simulink library "soar_lib"  (R2018b)
settings: Solver=VariableStepAuto  StartTime=0.0  StopTime=10.0  RelTol=1e-3
settings Model: Creator=Taylor  LastModifiedBy=Taylor
settings SFSimCC: SimUseLocalCustomCode=off
settings RTWCC: RTWUseLocalCustomCode=off
settings CodeAppCC: StateflowObjectComments=on

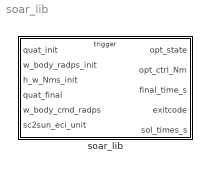
== system soar_lib ==
  soar_lib : Subsystem

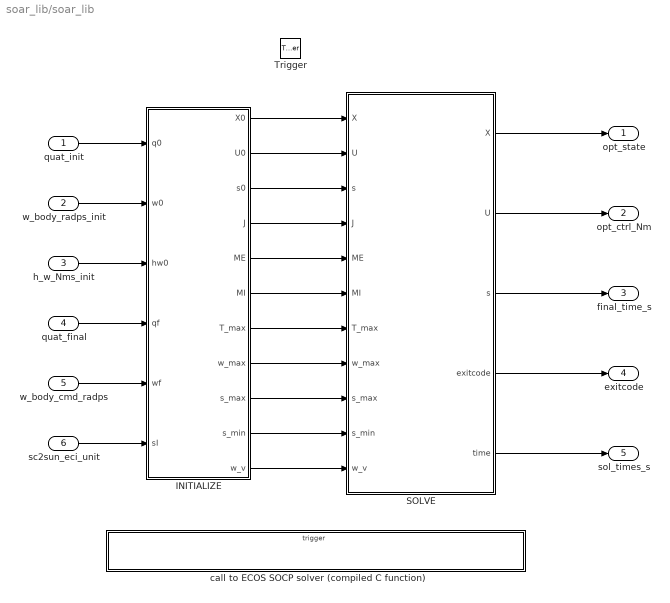
== system soar_lib/soar_lib ==
  quat_init : Inport
  w_body_radps_init : Inport  Port=2
  h_w_Nms_init : Inport  Port=3
  quat_final : Inport  Port=4
  w_body_cmd_radps : Inport  Port=5
  sc2sun_eci_unit : Inport  Port=6
  Trigger : TriggerPort  VariantControl=Variant  StatesWhenEnabling=reset  ZeroCross=off  InitialTriggerSignalState=zero  PortDimensions=1
  INITIALIZE : MATLAB Function  TreatAsAtomicUnit=on
  SOLVE : MATLAB Function  TreatAsAtomicUnit=on
  call to ECOS SOCP solver (compiled C function) : Subsystem  TreatAsAtomicUnit=on
  opt_state : Outport
  opt_ctrl_Nm : Outport  Port=2
  final_time_s : Outport  Port=3
  exitcode : Outport  Port=4
  sol_times_s : Outport  Port=5
  wires:
  h_w_Nms_init/1 -> INITIALIZE/3(hw0)
  sc2sun_eci_unit/1 -> INITIALIZE/6(sI)
  w_body_cmd_radps/1 -> INITIALIZE/5(wf)
  quat_final/1 -> INITIALIZE/4(qf)
  w_body_radps_init/1 -> INITIALIZE/2(w0)
  quat_init/1 -> INITIALIZE/1(q0)
  INITIALIZE/1(X0) -> SOLVE/1("X ")
  INITIALIZE/11(w_v) -> SOLVE/11(w_v)
  INITIALIZE/2(U0) -> SOLVE/2("U ")
  INITIALIZE/3(s0) -> SOLVE/3("s ")
  INITIALIZE/4(J) -> SOLVE/4(J)
  INITIALIZE/5(ME) -> SOLVE/5(ME)
  INITIALIZE/6(MI) -> SOLVE/6(MI)
  INITIALIZE/7(T_max) -> SOLVE/7(T_max)
  INITIALIZE/8(w_max) -> SOLVE/8(w_max)
  INITIALIZE/9(s_max) -> SOLVE/9(s_max)
  INITIALIZE/10(s_min) -> SOLVE/10(s_min)
  SOLVE/1(X) -> opt_state/1
  SOLVE/2(U) -> opt_ctrl_Nm/1
  SOLVE/3(s) -> final_time_s/1
  SOLVE/4(exitcode) -> exitcode/1
  SOLVE/5(time) -> sol_times_s/1

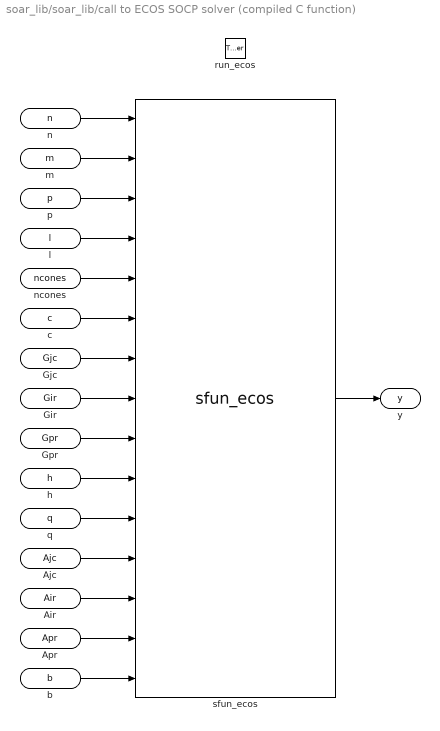
== system soar_lib/soar_lib/call to ECOS SOCP solver (compiled C function) ==
  run_ecos : TriggerPort  TriggerType=function-call  IsSimulinkFunction=on  FunctionName=run_ecos  FunctionVisibility=scoped  VariantControl=(inherit)
  sfun_ecos : S-Function  FunctionName=sfun_ecos  SFunctionDeploymentMode=off  EnableBusSupport=off  mask(Legacy Function){}
      mask help:
      | This block allows you to call the legacy functions specified by the following Legacy Code Tool definition:
      | def.SFunctionName = 'sfun_ecos';
      | def.OutputFcnSpec = 'solve_simple_optimization(int32 p1,int32 p2,int32 p3,int32 p4,int32 p5,double p6[18],int32 p7[19],int32 p8[57],double u1[57],double u2[38],int32 p9[6],int32 p10[19],int32 p11[16],double u3[16],double u4[6],solution y1[1])';
      | def.HeaderFiles = {'ecos.h', 'matlab_header.h'};
      | def.SourceFiles = {'main.c', 'cone.c', 'ctrlc.c', 'ecos.c', 'equil.c', 'expcone.c', 'kkt.c', 'preproc.c', 'spla.c', 'splamm.c', 'timer.c', 'wright_omega.c', 'ldl.c', 'amd_1.c', 'amd_2.c', 'amd_aat.c', 'amd_control.c', 'amd_defaults.c', 'amd_dump.c', 'amd_global.c', 'amd_info.c', 'amd_order.c', 'amd_post_tree.c', 'amd_postorder.c', 'amd_preprocess.c', 'amd_valid.c'};
      | def.IncPaths = {'./ecos/include', './ecos/external/ldl/include', './ecos/external/amd/include', './ecos/external/SuiteSparse_config'};
      | def.SrcPaths = {'./ecos/src', './ecos/external/ldl/src', './ecos/external/amd/src'};
      mask Help: <p>This block was generated automatically by the Legacy Code Tool. For detailed help on this tool, call<a href="matlab:legacy_code('help')"> legacy_code('help')</a>.</p>
      mask DialogControl DescTextVar Prompt: <b>Mathematical Description of SOAR</b><br><br>  Computes one solve step of the optimal attitude reorientation problem by solving a minimum-time constrained attitute control problem via convex optimization. Formulation: <br> <br> min c'*z<br>subject to<br>A*z=b<br>G*z&lt;=_K h <br> <br> Where &lt;=_K denotes a generalized inequality with respect to the cone K, i.e. the vector h-G*z belongs to the cone K. The cone K may be an n-dimensional positive orthant (R_+^n, which simply means G*z &lt;=h is the usual inequality) or a second-order Q^n defined as: <br> <br> Q^n = {(t(z),x(z)) in R x R^{n-1} | t(z) &lt;= ||x(z)||_2} <br> <br> For the latter case, h-G*z defines then the (t,x) in R^n vector. The case of exponential cones, which ECOS can handle, does not appear in the attitude control problem problem and is not considered here.<br><br> <b>ECOS C API</b><br><br> n : Number of primal variables<br> m : Number of generalized inequality constraints, i.e. dimension 1 of matrix G and length of vector h<br> p : Number of equality constraints, i.e. dimension 1 of matrix A and length of vector b<br> l : Dimension of the positive orthan R_+^l (number of usual inequality constraints)<br> ncones : Number of second-order cones<br> q : Array of length ncones; q[i] defines the dimension of the cone i<br> Gpr, Gjc, Gir : Arrays of matrix G in column compressed storage (CCS)<br> Apr, Ajc, Air : Arrays of matrix A in column compressed storage (CCS)<br> c : Array of length n (cost)<br> h : Array of length m (RHS of generalized inequality constraints)<br> b : Array of length p (RHS of equality constraints)<br>
      mask Display:
      | %%% Input port labels
      | port_label('input',1,'n');
      | port_label('input',2,'m');
      | port_label('input',3,'p');
      | port_label('input',4,'l');
      | port_label('input',5,'ncones');
      | port_label('input',6,'c');
      | port_label('input',7,'Gjc');
      | port_label('input',8,'Gir');
      | port_label('input',9,'Gpr');
      | port_label('input',10,'h');
      | port_label('input',11,'q');
      | port_label('input',12,'Ajc');
      | port_label('input',13,'Air');
      | port_label('input',14,'Apr');
      | port_label('input',15,'b');
      | %%% Outputs port labels
      | port_label('output',1,'optimal_solution');
  n : ArgIn  DisableCoverage=on  OutDataTypeStr=int32  ArgumentName=n
  m : ArgIn  DisableCoverage=on  Port=2  OutDataTypeStr=int32  ArgumentName=m
  p : ArgIn  DisableCoverage=on  Port=3  OutDataTypeStr=int32  ArgumentName=p
  l : ArgIn  DisableCoverage=on  Port=4  OutDataTypeStr=int32  ArgumentName=l
  ncones : ArgIn  DisableCoverage=on  Port=5  OutDataTypeStr=int32  ArgumentName=ncones
  c : ArgIn  DisableCoverage=on  Port=6  PortDimensions=soarParams.c_size  ArgumentName=c
  Gjc : ArgIn  DisableCoverage=on  Port=7  OutDataTypeStr=int32  PortDimensions=soarParams.Gjc_size  ArgumentName=Gjc
  Gir : ArgIn  DisableCoverage=on  Port=8  OutDataTypeStr=int32  PortDimensions=soarParams.Gir_size  ArgumentName=Gir
  Gpr : ArgIn  DisableCoverage=on  Port=9  PortDimensions=soarParams.Gpr_size  ArgumentName=Gpr
  h : ArgIn  DisableCoverage=on  Port=10  PortDimensions=soarParams.h_size  ArgumentName=h
  q : ArgIn  DisableCoverage=on  Port=11  OutDataTypeStr=int32  PortDimensions=soarParams.q_size  ArgumentName=q
  Ajc : ArgIn  DisableCoverage=on  Port=12  OutDataTypeStr=int32  PortDimensions=soarParams.Ajc_size  ArgumentName=Ajc
  Air : ArgIn  DisableCoverage=on  Port=13  OutDataTypeStr=int32  PortDimensions=soarParams.Air_size  ArgumentName=Air
  Apr : ArgIn  DisableCoverage=on  Port=14  PortDimensions=soarParams.Apr_size  ArgumentName=Apr
  b : ArgIn  DisableCoverage=on  Port=15  PortDimensions=soarParams.b_size  ArgumentName=b
  y : ArgOut  DisableCoverage=on  PortDimensions=soarParams.y_size  ArgumentName=y
  wires:
  sfun_ecos/1 -> y/1
  n/1 -> sfun_ecos/1
  m/1 -> sfun_ecos/2
  p/1 -> sfun_ecos/3
  l/1 -> sfun_ecos/4
  ncones/1 -> sfun_ecos/5
  Gjc/1 -> sfun_ecos/7
  Gir/1 -> sfun_ecos/8
  q/1 -> sfun_ecos/11
  Ajc/1 -> sfun_ecos/12
  Air/1 -> sfun_ecos/13
  c/1 -> sfun_ecos/6
  Gpr/1 -> sfun_ecos/9
  h/1 -> sfun_ecos/10
  Apr/1 -> sfun_ecos/14
  b/1 -> sfun_ecos/15

== matlab function soar_lib/INITIALIZE ==
  data: q0 input size=4; w0 input size=3; hw0 input size=3; qf input size=4; wf input size=3; sI input size=3; X0 output; U0 output; s0 output; J output; ME output; MI output; T_max output; w_max output; s_max output; s_min output; w_v output; soarParams parameter
function [X0,U0,s0,J,ME,MI,T_max,w_max,s_max,s_min,w_v] = init_SOAR(q0,w0,hw0,qf,wf,sI,soarParams)
%INIT_SOAR    
%
% SOAR's init function. Initializes all parameters are provides the initial
% guess to SOAR's main solve function. 
%
% T. Reynolds -- RAIN Lab

%#codegen

% constraints
cB      = [ 0.0; 0.0; -1.0 ];   % camera boresight vector
ssB     = [ 0.0; 1.0; 0.0 ];    % sun sensor boresight vector
amin    = deg2rad(50);          % min. separating angle
amax    = deg2rad(60);          % FOV of sun sensor
Me      = [ sI'*cB             (skew(sI)*cB)';
            skew(sI)*cB  sI*cB'+cB*sI'-(sI'*cB)*eye(3) ] - cos(amin)*eye(4);
Mi      = [ sI'*ssB             (skew(sI)*ssB)';
            skew(sI)*ssB  sI*ssB'+ssB*sI'-(sI'*ssB)*eye(3) ] - cos(amax)*eye(4);
Met     = Me + 2*eye(4);    % M_exclude_tilde
Mit     = 2*eye(4) - Mi;    % M_include_tilde
% compute matrix square root. Cannot use MX = sqrtm(Mxt) since complex
% values may be returned, and these must be turned off for code generation
[Ve,De] = schur(Met);
[Vi,Di] = schur(Mit);
for k = 1:4
    De(k,k) = realsqrt(De(k,k));
    Di(k,k) = realsqrt(Di(k,k));
end
ME  = Ve*De*Ve';    % exclusion constraint matrix
MI  = Vi*Di*Vi';    % inclusion constraint matrix
s_min   = soarParams.s_min;       % min allowable time
s_max   = soarParams.s_max;       % max allowable time

% controller parameters
N       = 10;   % number of time nodes
Nx      = 10;   % number of states
Nu      = 3;    % number of controls

% spacecraft inertia matrix & constraint values (set in init_soac_params)
J       = soarParams.inertia;  % kg m2
T_max   = soarParams.T_max;    % mNm
w_max   = soarParams.w_max;    % rad/s
w_v     = soarParams.w_v;      % virtual control weight

% Initial trajectory
x0  = zeros(Nx,N);
u0  = zeros(Nu,N);
s0  = s_max; 
tau = linspace(0,1,N);
[qb,flag] = Q_SLERP(q0,qf);
if ( flag == 0 )
    for k = 1:N
        wk = zeros(3,1);
        for i = 1:3
           wk(i) = interp1([0 1],[w0(i) wf(i)],tau(k),'linear');
        end
        x0(:,k)   = [ qb(:,k); J*wk; hw0 ];
        u0(:,k)     = zeros(3,1);
    end
end

% Initial state and control guess
X0   = reshape(x0,Nx*N,1);
U0   = reshape(u0,Nu*N,1);

end

function [qt,FLAG] = Q_SLERP( q0,q1 )
%Q_SLERP 
%
% Q_SLERP(q0,q1,tspan) Uses Spherical Linear intERPolation to 
% interpolate between two quaternions given the time space tspan. 
% Both q0 and q1 must be quaternions.
%
% T.Reynolds -- RAIN Lab.
%#codegen

N    = 10;
FLAG = int8(0);

if ( length(q0)~=4 || length(q1)~=4 )
   FLAG = int8(1);
   qt   = repmat([1.0;0.0;0.0;0.0],1,N);
   return;
end

% Reshape inputs to be column vectors
q0  = reshape(q0, 4, 1);
q1  = reshape(q1, 4 ,1);

% Find angle between inputs -- careful to avoid degenerate numerical cases
% that lead to acos being imaginary.
temp = dot(q0,q1);
if (1.0-temp<0)
    ang = 0.0;
else
    ang = acos(temp);
end
if ( ang > pi )
    FLAG = int8(2);
    qt   = repmat([1.0;0.0;0.0;0.0],1,N);
    return;
end

sang = sin(ang);
% if sang is zero, then q0 and q1 are the same, and this will output q0 
if (sang<1e-8)
    qt = repmat(q0,1,N);
else
    qt   = zeros(4,N);
    for k = 1:N
        t       = (k-1)/(N-1);
        qt(:,k) = (sin((1 - t)*ang)/sang).*q0 + (sin(t*ang)/sang).*q1;
    end
end
end

== matlab function soar_lib/SOLVE ==
  data: X input; U input; s input; J input; ME input; MI input; T_max input; w_max input; s_max input; s_min input; w_v input; X output; soarParams parameter; U output; s output; exitcode output; time output
function [X,U,s,exitcode,time] = solve_SOAR(X,U,s,J,ME,MI,T_max,w_max,...
                        s_max,s_min,w_v,soarParams)                  
%                         c_size, Air_size, Ajc_size, Apr_size, b_size, ...
%                         Gir_size, Gjc_size, Gpr_size, h_size, q_size)
%SOLVE_SOAR     
%
% SOAR's main function that solves the problem fully.
%
% T. Reynolds -- RAIN Lab

%#codegen

N  = 10;        % number of time nodes
Nx = 10;        % number of states
Nu = 3;         % number of controls
iter_max = 15;  % maximum global iterations
config = soarParams.config;

% Get problem sizes
c_size   = soarParams.c_size;
b_size   = soarParams.b_size;
h_size   = soarParams.h_size;
q_size   = soarParams.q_size;
Air_size = soarParams.Air_size;
Ajc_size = soarParams.Ajc_size;
Apr_size = soarParams.Apr_size;
Gir_size = soarParams.Gir_size;
Gjc_size = soarParams.Gjc_size;
Gpr_size = soarParams.Gpr_size;
l_dim    = soarParams.l_dim;
soc_dim  = soarParams.soc_dim;
n        = c_size;     % primal variables
m        = h_size;     % number of inequality constraints
p        = b_size;     % number of equality constraints
l        = l_dim;      % dimension of linear cone
ncones   = q_size;     % number of SOCs
q        = soc_dim;    % dimension(s) of the SOCs
exitcode = zeros(iter_max+2,1);
time     = zeros(iter_max,1);

% Scaling matrices
% Dx  = soarParams.Dx;
% Du  = soarParams.Du;
% Ds  = soarParams.Ds;
% iDx = soarParams.iDx;

% Initial and final conditions stored in initial guess X
xi = X(1:Nx);
xf = X(Nx*(N-1)+(1:7)); % LEAVE THIS AS 7

for k = 1:iter_max
    
    % discretize
    [EH,BE,ES,AR] = foh(X,U,s,N,Nx,Nu,J);%,Dx,Du,Ds,iDx);
    
    % parse for ECOS
    [c,G,h,A,b] = parse_ecos(xi,xf,J,EH,BE,ES,AR,N,...
                             ME,MI,T_max,w_max,s_max,s_min,...
                             w_v,config);%,Dx,Du,Ds,iDx,config);
    
    % put A and G in compressed column storage
    [Air,Ajc,Apr] = convert_to_CCS(A,Air_size);
    [Gir,Gjc,Gpr] = convert_to_CCS(G,Gir_size);
           
    % call to ECOS
    y = run_ecos(n,m,p,l,ncones,c(1:c_size),...
                    Gjc(1:Gjc_size),Gir(1:Gir_size),Gpr(1:Gpr_size),...
                    h(1:h_size),reshape(q(1:q_size),q_size,1),...
                    Ajc(1:Ajc_size),Air(1:Air_size),Apr(1:Apr_size),...
                    b(1:b_size));
    
    % update solution
    diff        = norm(X - y(1:N*Nx),1); % difference in state vector
    X           = y(1:N*Nx); % soarParams.DX*y(1:N*Nx);
    U           = y(N*Nx+1:N*(Nx+Nu)); % soarParams.DU*y(N*Nx+1:N*(Nx+Nu));
    s           = y(N*(Nx+Nu)+2); % Ds*y(N*(Nx+Nu)+2);
    V           = y(N*(Nx+Nu)+3:N*(2*Nx+Nu)+1);
    exitcode(k) = y(c_size+1);
    time(k)     = y(c_size+2);
    % if one of the exitcodes indicates failue, the final
    % entry in exitcode is set to -1 to indicate this, and the
    % solution should not be used
    if (exitcode(k) ~= 0)
        exitcode(iter_max+2) = -1;
    end
    
    % check convergence. Note that we MUST take at least two iterations,
    % this is to avoid exiting early for very small maneuvers before things
    % have truly converged.
    if ( (k>1) && (norm(V,1) < 1e-5) && (diff < 5e-2) )
        % exit for loop since we've converged
        exitcode(iter_max+1) = k;
        break;
    end
            
end

% Sanity checks on the solution if we hit the max iterations
if (k==iter_max) % hit max global iterations
    exitcode(iter_max+1) = iter_max;
    if (exitcode(iter_max+2) ~= -1 )
        if (norm(V,1) > 1e-5)
            exitcode(iter_max+2) = 3; % does not clash with ECOS exitcodes
        elseif (diff>5e-2)
            exitcode(iter_max+2) = 4;
        end
    end
end

end

%%%%%%%%%%%%%%%%%%%%%%%%%%%%%%%%%%%%%%%%%%%%%%%%%%%%%%%%%%%%%%%%%%%%%%%%%%%
%%%%%%%%%%%%%%%%%%%%%%%%%%%% SUPPORT FUNCTIONS %%%%%%%%%%%%%%%%%%%%%%%%%%%%
%%%%%%%%%%%%%%%%%%%%%%%%%%%%%%%%%%%%%%%%%%%%%%%%%%%%%%%%%%%%%%%%%%%%%%%%%%%

function [ EH,BE,ES,AR ] = foh( X,U,s,N,Nx,Nu,J) %,Dx,Du,Ds,iDx )
%FOH   first order hold discretization
%
% FOH(X,U,s,N,Nx,Nu,J,Dx,Du,Dx) Computes the matrices (A,B,S,Z) 
% to numerically discretize a problem instance of SOAC about the trajectory 
% stored in X and U. Assumes a linear interpolation of the torque 
% between control nodes, of which there are N.
%
% These matrices give the first order Taylor series of the dynamics
% at the N time nodes dictated and correspond to a discrete time
% LTV system approximating the nonlinear dynamics.
%
% Inputs: 
%   - X (N*Nx by 1) current state at each discrete node
%   - U (N*Nu by 1) current control at each discrete node
%   - s (1 by 1) current final time
%   - N (1 by 1) number of discrete time nodes
%   - Nx (1 by 1) number of states
%   - Nu (1 by 1) number of controls
%   - J (3 by 3) spacecraft inertia matrix
%   - [omitted] Dx (Nx by Nx) scaling matrix for the state
%   - [omitted] Du (Nu by Nu) scaling matrix for the control
%   - [omitted] Ds (1 by 1) scaling matrix for the final time
%   - [omitted] iDx (Nx by Nx) inverse of Dx, precomputed
% Outputs: 
%   - EH (N*Nx by N*Nx)
%   - BE (N*Nu by N*Nu)
%   - ES (N*Nx by 1)
%   - ZE (N*Nx by 1)
%
% T. Reynolds -- RAIN Lab
%#codegen

len     = N-1;              % number of transition matrices
tau     = linspace(0,1,N);  % normalized time
Nsub    = 10;               % number of sub-interval points

% Set sizes for each discrete matrix
EH          = zeros(Nx*(len+1),Nx*(len+1));
EH(1:Nx,1:Nx) = eye(Nx);
BE          = zeros(Nx*(len+1),Nu*(len+1));
ES          = zeros(Nx*(len+1),1);
AR          = zeros(Nx*(len+1),1);

% Initial conditions
A0  = eye(Nx);
B0p = zeros(Nx*Nu,1);
B0m = zeros(Nx*Nu,1);
S0  = zeros(Nx,1);
R0  = zeros(Nx,1);

for k = 1:len
    
    % (re)define initial condition for integration
    xF = X(Nx*(k-1)+(1:Nx));
    P0 = [xF(:); A0(:); B0p(:); B0m(:); S0(:); R0(:)];
    
    um = U(Nu*(k-1)+(1:Nu));
    up = U(Nu*k+(1:Nu));
    u  = [reshape(um,Nu,1) reshape(up,Nu,1)];
    tspan = linspace(tau(k), tau(k+1), N);
    
    for k_ = 1:Nsub-1
        
        tk      = tspan(k_);
        tkp1    = tspan(k_+1);
        h       = tkp1-tk;
        
        k1 = deriv(tk    ,P0       ,u,tspan,s,J);
        k2 = deriv(tk+h/2,P0+h/2*k1,u,tspan,s,J);
        k3 = deriv(tk+h/2,P0+h/2*k2,u,tspan,s,J);
        k4 = deriv(tk+h  ,P0+h*k3  ,u,tspan,s,J);
        
        P0 = (P0+h/6*(k1+2*k2+2*k3+k4));
    end
    
    AF  = P0(Nx+1:Nx*(Nx+1));
    BFp = P0(Nx*(Nx+1)+1:Nx*(Nx+Nu+1));
    BFm = P0(Nx*(Nx+Nu+1)+1:Nx*(Nx+2*Nu+1));
    SF  = P0(Nx*(Nx+2*Nu+1)+1:Nx*(Nx+2*Nu+2));
    RF  = P0(Nx*(Nx+2*Nu+2)+1:Nx*(Nx+2*Nu+3));
    
    % Fill up matrices
    Ad  = reshape(AF,Nx,Nx);
    EH(Nx*k+(1:Nx),Nx*(k-1)+(1:Nx)) = Ad; % iDx*Ad*Dx;
    BE(Nx*k+(1:Nx),Nu*(k-1)+(1:Nu)) = Ad*reshape(BFm,Nx,Nu); % iDx*(Ad*reshape(BFm,Nx,Nu))*Du;
    BE(Nx*k+(1:Nx),Nu*k+(1:Nu))     = Ad*reshape(BFp,Nx,Nu); % iDx*(Ad*reshape(BFp,Nx,Nu))*Du;
    ES(Nx*k+(1:Nx))                 = Ad*reshape(SF,Nx,1); % iDx*(Ad*reshape(SF,Nx,1))*Ds;
    AR(Nx*k+(1:Nx))                 = Ad*reshape(RF,Nx,1); % iDx*Ad*reshape(RF,Nx,1);
    
end


end

function DX = deriv(t,X,u,tspan,s,J)
%#codegen
    Nx = 10;
    x   = X(1:Nx); 
    
    [f,A,Bp,Bm,Z] = get_f_vals(t,x,u,tspan,J);
    
    Phi = reshape(X(Nx+1:Nx*(Nx+1)),size(A));
       
    xdot        = s*f;
    Phi_dot     = (s*A)*Phi;
    Bdp_dot     = Phi\(s*Bp);
    Bdm_dot     = Phi\(s*Bm);
    Sd_dot      = Phi\f;
    Zd_dot      = Phi\(s*Z);
    
    DX      = [ xdot(:); Phi_dot(:); Bdp_dot(:);...
                Bdm_dot(:); Sd_dot(:); Zd_dot(:)];
end

function [f,A,Bp,Bm,Z] = get_f_vals(t,x,u,tspan,J)
%#codegen   
    tkm     = tspan(1);
    tkp     = tspan(end);     
    lam_km  = (tkp - t)/(tkp - tkm);
    lam_kp  = (t - tkm)/(tkp - tkm);
    
    % Interpolate u
    u_tau = lam_km .* u(:,1) + lam_kp .* u(:,2);

    % compute jacobian matrices
    [A,B,f] = Q_linearize(t,x,u_tau,J);
    
    Bp  = lam_kp*B;
    Bm  = lam_km*B;
    
    % compute z
    Z   = - A*x - B*u_tau;
                           
end

function [ A,B,f ] = Q_linearize( t,x,u,J )
%Q_LINEARIZE    Linearize the attitude dynamics
%
% Q_linearize(t,x,u,P) returns the discrete representation of the
% quaternion-based attitude dynamics at the point (x,u) and time t.
%
% T. Reynolds -- RAIN Lab.
%#codegen

% States
q   = x(1:4)./norm(x(1:4));
q0  = q(1);
qv  = q(2:4);
hb  = x(5:7);
hw  = x(8:10);
w   = J\hb;

% Partials
dfq_dq      = 0.5 * [ 0 -w'; w -skew(w) ];
dfq_dhb     = 0.5 * [ -qv'; skew(qv)+q0*eye(3) ]/J;
dfq_dhw     = zeros(4,3);
dfhb_dq     = zeros(3,4);
dfhb_dhb    = skew(hb)/J - skew(w) + skew(hw)/J;
dfhb_dhw    = -skew(w);
dfhw_dq     = zeros(3,4);
dfhw_dhb    = zeros(3,3);
dfhw_dhw    = zeros(3,3);
dfq_du      = zeros(4,3);
dfhb_du     = -eye(3);
dfhw_du     = eye(3);

% Kinematics & Dynamics
fq  = 0.5 * [ -qv'; skew(qv)+q0*eye(3) ] * w;
fhb = -u + skew(hb+hw)*w;
fhw = u;

% Outputs
f = [ fq; fhb; fhw ];
A = [ dfq_dq dfq_dhb dfq_dhw;
      dfhb_dq dfhb_dhb dfhb_dhw;
      dfhw_dq dfhw_dhb dfhw_dhw ];
B = [ dfq_du; dfhb_du; dfhw_du ];

end

function [c,G,h,A,b] = parse_ecos(xi,xf,J,EH,BE,ES,AR,N,...
                                  ME,MI,T_max,w_max,s_max,s_min,...
                                  w_v,config)%,Dx,Du,Ds,iDx,config)
%#codegen
u_max = T_max .* ones(N*3,1);
w_max = w_max .* ones(N*3,1);
Nx = 10;
Nu = 3;
% Dq = Dx(1:4,1:4); % this is identity, so ignoring for now
% Dw = Dx(5:7,5:7);

% Hw  = [ kron(eye(N),[zeros(3,4) inv(J) zeros(3)]*Dx) ...
%         zeros(3*N,N*(Nu+2*Nx)+2) ];
Hw  = [ kron(eye(N),[zeros(3,4) inv(J) zeros(3)]) ...
        zeros(3*N,N*(Nu+2*Nx)+2) ];
% Hu  = [ zeros(N*3,N*Nx) kron(eye(N),eye(Nu)*Du) zeros(N*3,2*N*Nx+2) ];
Hu  = [ zeros(N*3,N*Nx) kron(eye(N),eye(Nu)) zeros(N*3,2*N*Nx+2) ];
Hv  = [ zeros(N*Nx) zeros(N*Nx,N*3) ...
        zeros(N*Nx,2) eye(N*Nx) zeros(N*Nx,N*Nx) ];
Hg  = [ zeros(1,N*(Nx+3)) 1 0 zeros(1,2*N*Nx) ];
% Hs  = [ zeros(1,N*(Nx+3)) 0 Ds zeros(1,2*N*Nx) ];
Hs  = [ zeros(1,N*(Nx+3)) 0 1 zeros(1,2*N*Nx) ];
Hev = [ zeros(N*Nx,N*(2*Nx+3)+2) eye(N*Nx) ];

% Cost function
c = [ zeros(N*(Nx+Nu),1); 1; 0; zeros(N*Nx,1); w_v*ones(N*Nx,1) ];
% Equality constraints
% A = [ eye(Nx) repmat(zeros(Nx),1,N-1) zeros(Nx,N*(Nu+2*Nx)+2);
%     EH-eye(size(EH)) BE zeros(N*Nx,1) ES kron(eye(N),iDx) zeros(N*Nx,N*Nx);
%     repmat(zeros(7,Nx),1,N-1) horzcat(blkdiag(eye(4),Dw),zeros(7,3)) ...
%     zeros(7,N*(Nu+2*Nx)+2) ];
A = [ eye(Nx) repmat(zeros(Nx),1,N-1) zeros(Nx,N*(Nu+2*Nx)+2);
    EH-eye(size(EH)) BE zeros(N*Nx,1) ES eye(N*Nx) zeros(N*Nx,N*Nx);
    repmat(zeros(7,Nx),1,N-1) horzcat(eye(7),zeros(7,3)) ...
    zeros(7,N*(Nu+2*Nx)+2) ];
b = [xi; -AR; xf];
% Inequality constraints
Glin    = [ Hw; -Hw; Hu; -Hu; Hs; -Hs; Hv-Hev; -Hv-Hev ];
hlin    = [ w_max; w_max; u_max; u_max; ...
            s_max; -s_min; zeros(N*Nx,1); zeros(N*Nx,1) ];
% if (strcmp(config,'bie'))
%     Gquad = zeros(152,332);
%     hquad = zeros(152,1);
% elseif (strcmp(config,'bi'))
%     Gquad = zeros(92,332);
%     hquad = zeros(92,1);
% else
%     Gquad = zeros(32,332);
%     hquad = zeros(32,1);
% end
Gquad   = [ -Hg./sqrt(2); -Hu; Hg./sqrt(2) ];
hquad   = [ 1/sqrt(2); zeros(size(Hu,1),1); 1/sqrt(2) ];
if (strncmp(config,'bi',2))
    Hq  = [ eye(4) zeros(4,6) ];
    Gquad_ = [Gquad; zeros(60,332)];
    hquad_ = [hquad; zeros(60,1)];
    for k = 1:N
        Hk = zeros(Nx,332);
        Hk(1:Nx,Nx*(k-1)+(1:Nx)) = eye(Nx);
%         Pk = MI*Hq*Dx*Hk;
        Pk = MI*Hq*Hk;
        Gk = [ zeros(1,332); -Pk; zeros(1,332) ];
        hk = [ 3/sqrt(2); zeros(size(Pk,1),1); -1/sqrt(2) ];
        Gquad_(6*(k-1)+(33:38),:) = Gk;
        hquad_(6*(k-1)+(33:38)) = hk;
    end
    if (strcmp(config,'bie'))
        Gquad__ = [Gquad_; zeros(60,332)];
        hquad__ = [hquad_; zeros(60,1)];
        for k = 1:N
            Hk = zeros(Nx,332);
            Hk(1:Nx,Nx*(k-1)+(1:Nx)) = eye(Nx);
%             Pk = ME*Hq*Dx*Hk;
            Pk = ME*Hq*Hk;
            Gk = [ zeros(1,332); -Pk; zeros(1,332) ];
            hk = [ 3/sqrt(2); zeros(size(Pk,1),1); -1/sqrt(2) ];
            Gquad__(6*(k-1)+(33:38),:) = Gk;
            hquad__(6*(k-1)+(33:38)) = hk;
        end
        G = [Glin;Gquad__];
        h = [hlin;hquad__];
    else
        G = [Glin;Gquad_];
        h = [hlin;hquad_];
    end
else
    G = [Glin;Gquad];
    h = [hlin;hquad];
end    

end % parse_ecos

function [Xir,Xjc,Xpr] = convert_to_CCS(X,Xir_size)
%#codegen
    [Xir,Xpr] = my_find(X,Xir_size);
    Xjc = zeros(size(X,2)+1,1,'int32');
    for col = 2:size(X,2)
        Xjc(col) = Xjc(col-1)+int32(nnz(X(:,col-1)));
    end
    Xjc(end) = int32(nnz(X));
end

function [Xir,Xpr] = my_find(X,Xir_size)
%#codegen
% [n,m] = size(X);
n = int32(size(X,1));
m = int32(size(X,2));
Xir   = zeros(Xir_size,1,'int32');
Xpr   = zeros(Xir_size,1);
X_nnz = nnz(X);
id = 1;
for col = 1:m
    for row = 1:n
        if ((X(row,col)~=0) && (id<X_nnz+1))
            Xir(id) = row-1; % zero based row indexing
            Xpr(id) = X(row,col);
            id = id + 1;
        end
    end
end
end

% function [ Mir,Mjc,Mpr ] = convert_to_CCS( M )
% %#codegen
% [Mir,~,Mpr] = find(M);
% Mir = Mir - 1; % CCS uses zero-based row indexing
% Mjc = zeros(size(M,2)+1,1);
% for col = 2:size(M,2)
%     Mjc(col) = Mjc(col-1)+nnz(M(:,col-1));
% end
% Mjc(end) = length(find(M~=0));
% 
% end
